simulink library "sm_trackV_lib_terrain_contact_s46"  (R2026a)
settings: Solver=VariableStepAuto
undefined symbols (not defined in the file): B1, B2, B3, B4, B5, B6, B7, B8, L1, L10, L11, L12, L13, L14, L15, L16, L17, L18, L19, L2, L20, L21, L22, L23, L24, L25, L26, L27, L28, L29, L3, L30, L31, L32, L33, L34, L35, L36, L37, L38, L39, L4, L40, L41, L42, L43, L44, L45, L46, L5, L6, L7, L8, L9, Road, Scene, X, Y, Z
libraries: sm_trackV_lib_terrain_contact_elem x92, $bdroot x22, sm_excv_scene_lib x5, sm_lib x4
Description:
  | Copyright 2024-2026 The MathWorks, Inc.
settings Model: Creator=smiller  LastModifiedBy=smiller

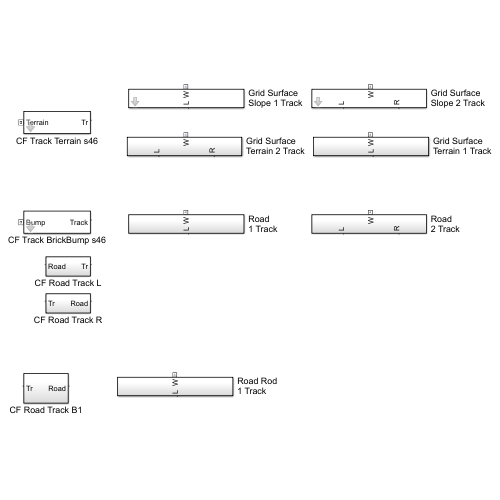
[thumbnail: Simulink's stored preview of the top-level diagram]
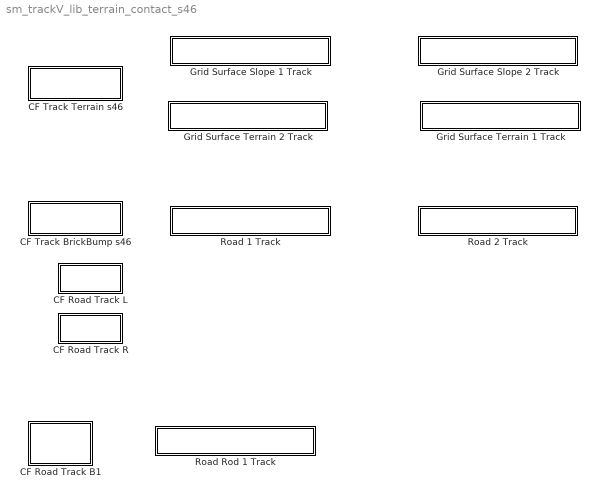
== system sm_trackV_lib_terrain_contact_s46 ==
  CF Road Track B1 : Subsystem
  CF Road Track L : Subsystem
  CF Road Track R : Subsystem
  CF Track BrickBump s46 : Subsystem  mask(Contact Forces, Full Track to Bump){K_BrickBump=Scene.Contact.BrickBump.K, B_BrickBump=Scene.Contact.BrickBump.B, TW_BrickBump=Scene.Contact.BrickBump.TW}
      mask prompts: K_BrickBump "Normal Stiffness (N/m)"; B_BrickBump "Normal Damping (N/(m/s))"; TW_BrickBump "Normal Transition Width (m)"
      mask help: Models contact force between all track segments and bump.
  CF Track Terrain s46 : Subsystem  mask(Contact Forces, Full Track to Terrain){K_Road=Scene.Contact.Terrain.K, B_Road=Scene.Contact.Terrain.B, TW_Road=Scene.Contact.Terrain.TW, F_dyn_Road=Scene.Contact.Terrain.mud, F_stat_Road=Scene.Contact.Terrain.mus, CV_Road=Scene.Contact.Terrain.CV}
      mask prompts: K_Road "Normal Stiffness (N/m)"; B_Road "Normal Damping (N/(m/s))"; TW_Road "Normal Transition Width (m)"; F_dyn_Road "Coefficient of Dynamic Friction"; F_stat_Road "Coefficient of Static Friction"; CV_Road "Critical Velocity (m/s)"
      mask help: Models contact force between all track segments and the terrain.
  Grid Surface Slope 1 Track : Subsystem  mask{road_len=Scene.Slope.road_len, road_wid=Scene.Slope.road_wid, slope_rise=Scene.Slope.slope_rise, slope_run=Scene.Slope.slope_run, slope_x0=Scene.Slope.slope_start, slope_xres=Scene.Slope.slope_xres, surface_clr=Scene.Slope.clr, surface_opc=Scene.Slope.opc, K_Road=Scene.Contact.Terrain.K, B_Road=Scene.Contact.Terrain.B, TW_Road=Scene.Contact.Terrain.TW, F_dyn_Road=Scene.Contact.Terrain.mud, F_stat_Road=Scene.Contact.Terrain.mus, CV_Road=Scene.Contact.Terrain.CV}
      mask prompts: road_len "Road Length (m)"; road_wid "Road Width (m)"; slope_rise "Slope Rise (m)"; slope_run "Slope Run(m)"; slope_x0 "Slope Start (m)"; slope_xres "Slope Resolution (m)"; surface_clr "Color [R G B] (0-1)"; surface_opc "Opacity (0-1)"; K_Road "Normal Stiffness (N/m)"; B_Road "Normal Damping (N/(m/s))"; TW_Road "Normal Transition Width (m)"; F_dyn_Road "Coefficient of Dynamic Friction"; F_stat_Road "Coefficient of Static Friction"; CV_Road "Critical Velocity (m/s)"
      mask TypeOptions road_len:
      | Grid Surface
      | Slope/road_len
      mask TypeOptions road_wid:
      | Grid Surface
      | Slope/road_wid
      mask TypeOptions slope_rise:
      | Grid Surface
      | Slope/slope_rise
      mask TypeOptions slope_run:
      | Grid Surface
      | Slope/slope_run
      mask TypeOptions slope_x0:
      | Grid Surface
      | Slope/slope_x0
      mask TypeOptions slope_xres:
      | Grid Surface
      | Slope/slope_xres
      mask TypeOptions surface_clr:
      | Grid Surface
      | Slope/surface_clr
      mask TypeOptions surface_opc:
      | Grid Surface
      | Slope/surface_opc
      mask TypeOptions K_Road: CF Track Terrain L/K_Road
      mask TypeOptions B_Road: CF Track Terrain L/B_Road
      mask TypeOptions TW_Road: CF Track Terrain L/TW_Road
      mask TypeOptions F_dyn_Road: CF Track Terrain L/F_dyn_Road
      mask TypeOptions F_stat_Road: CF Track Terrain L/F_stat_Road
      mask TypeOptions CV_Road: CF Track Terrain L/CV_Road
      mask DialogControl cont_slope Prompt: Slope
      mask DialogControl cont_contact Prompt: Contact
  Grid Surface Slope 2 Track : Subsystem  mask{road_len=Scene.Slope.road_len, road_wid=Scene.Slope.road_wid, slope_rise=Scene.Slope.slope_rise, slope_run=Scene.Slope.slope_run, slope_x0=Scene.Slope.slope_start, slope_xres=Scene.Slope.slope_xres, surface_clr=Scene.Slope.clr, surface_opc=Scene.Slope.opc, TW_Road=Scene.Contact.Terrain.TW, B_Road=Scene.Contact.Terrain.B, K_Road=Scene.Contact.Terrain.K, F_dyn_Road=Scene.Contact.Terrain.mud, F_stat_Road=Scene.Contact.Terrain.mus, CV_Road=Scene.Contact.Terrain.CV}
      mask prompts: road_len "Road Length (m)"; road_wid "Road Width (m)"; slope_rise "Slope Rise (m)"; slope_run "Slope Run(m)"; slope_x0 "Slope Start (m)"; slope_xres "Slope Resolution (m)"; surface_clr "Color [R G B] (0-1)"; surface_opc "Opacity (0-1)"; TW_Road "Normal Transition Width (m)"; B_Road "Normal Damping (N/(m/s))"; K_Road "Normal Stiffness (N/m)"; F_dyn_Road "Coefficient of Dynamic Friction"; F_stat_Road "Coefficient of Static Friction"; CV_Road "Critical Velocity (m/s)"
      mask TypeOptions road_len:
      | Grid Surface
      | Slope/road_len
      mask TypeOptions road_wid:
      | Grid Surface
      | Slope/road_wid
      mask TypeOptions slope_rise:
      | Grid Surface
      | Slope/slope_rise
      mask TypeOptions slope_run:
      | Grid Surface
      | Slope/slope_run
      mask TypeOptions slope_x0:
      | Grid Surface
      | Slope/slope_x0
      mask TypeOptions slope_xres:
      | Grid Surface
      | Slope/slope_xres
      mask TypeOptions surface_clr:
      | Grid Surface
      | Slope/surface_clr
      mask TypeOptions surface_opc:
      | Grid Surface
      | Slope/surface_opc
      mask TypeOptions TW_Road: CF Track Terrain L/TW_Road | CF Track Terrain R/TW_Road
      mask TypeOptions B_Road: CF Track Terrain L/B_Road | CF Track Terrain R/B_Road
      mask TypeOptions K_Road: CF Track Terrain L/K_Road | CF Track Terrain R/K_Road
      mask TypeOptions F_dyn_Road: CF Track Terrain L/F_dyn_Road | CF Track Terrain R/F_dyn_Road
      mask TypeOptions F_stat_Road: CF Track Terrain L/F_stat_Road | CF Track Terrain R/F_stat_Road
      mask TypeOptions CV_Road: CF Track Terrain L/CV_Road | CF Track Terrain R/CV_Road
      mask DialogControl cont_slope Prompt: Slope
      mask DialogControl cont_contact Prompt: Contact
  Grid Surface Terrain 1 Track : Subsystem
  Grid Surface Terrain 2 Track : Subsystem
  Road 1 Track : Subsystem
  Road 2 Track : Subsystem
  Road Rod 1 Track : Subsystem

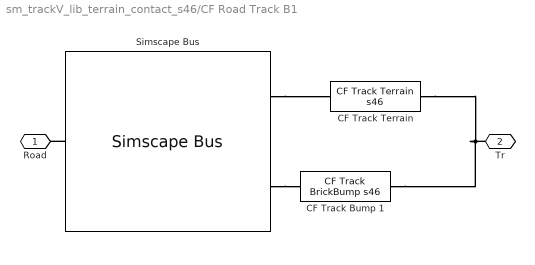
== system sm_trackV_lib_terrain_contact_s46/CF Road Track B1 ==
  CF Track Bump 1 : $bdroot/CF Track BrickBump s46  K_BrickBump=Scene.Contact.BrickBump.K  B_BrickBump=Scene.Contact.BrickBump.B  TW_BrickBump=Scene.Contact.BrickBump.TW
      settings: LibrarySourceBlock=sm_chain_drive_lib/CF_BrickBump_Full
  CF Track Terrain : $bdroot/CF Track Terrain s46  K_Road=Scene.Contact.Terrain.K  B_Road=Scene.Contact.Terrain.B  TW_Road=Scene.Contact.Terrain.TW  F_dyn_Road=Scene.Contact.Terrain.mud  F_stat_Road=Scene.Contact.Terrain.mus  CV_Road=Scene.Contact.Terrain.CV
      settings: LibrarySourceBlock=sm_chain_drive_lib/CF_Road_Full
  Simscape Bus : SimscapeBus  HierarchyStrings=Road;B1  ConnectionType=Bus: CBO_Road8
  Road : PMIOPort  Side=Left
  Tr : PMIOPort  Port=2  Side=Right
  connections:
  CF Track Terrain/RConn1 -- Tr/RConn1 -- CF Track Bump 1/RConn1
  Simscape Bus/RConn1 -- Road/RConn1
  Simscape Bus/LConn1 -- CF Track Terrain/LConn1
  Simscape Bus/LConn2 -- CF Track Bump 1/LConn1

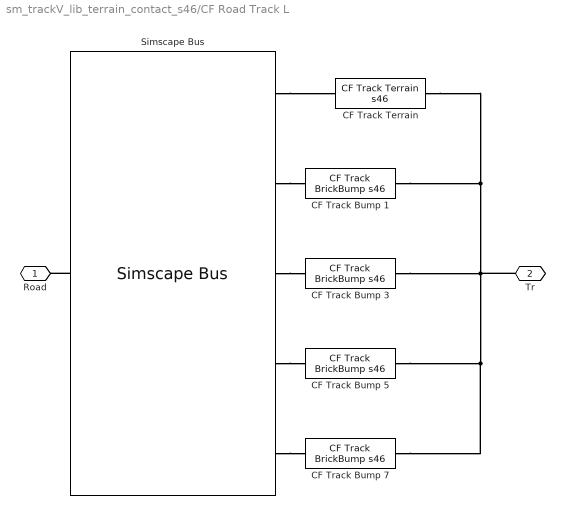
== system sm_trackV_lib_terrain_contact_s46/CF Road Track L ==
  CF Track Bump {1,3,5,7} (4 alike) : $bdroot/CF Track BrickBump s46  K_BrickBump=Scene.Contact.BrickBump.K  B_BrickBump=Scene.Contact.BrickBump.B  TW_BrickBump=Scene.Contact.BrickBump.TW
      settings: LibrarySourceBlock=sm_chain_drive_lib/CF_BrickBump_Full
  CF Track Terrain : $bdroot/CF Track Terrain s46  K_Road=Scene.Contact.Terrain.K  B_Road=Scene.Contact.Terrain.B  TW_Road=Scene.Contact.Terrain.TW  F_dyn_Road=Scene.Contact.Terrain.mud  F_stat_Road=Scene.Contact.Terrain.mus  CV_Road=Scene.Contact.Terrain.CV
      settings: LibrarySourceBlock=sm_chain_drive_lib/CF_Road_Full
  Simscape Bus : SimscapeBus  HierarchyStrings=Road;B1;B3;B5;B7  ConnectionType=Bus: CBO_Road8
  Road : PMIOPort  Side=Left
  Tr : PMIOPort  Port=2  Side=Right
  connections:
  Simscape Bus/LConn3 -- CF Track Bump 3/LConn1
  Simscape Bus/LConn2 -- CF Track Bump 1/LConn1
  Simscape Bus/LConn1 -- CF Track Terrain/LConn1
  Simscape Bus/RConn1 -- Road/RConn1
  Simscape Bus/LConn4 -- CF Track Bump 5/LConn1
  Simscape Bus/LConn5 -- CF Track Bump 7/LConn1
  CF Track Bump 1/RConn1 -- Tr/RConn1 -- CF Track Bump 7/RConn1 -- CF Track Bump 5/RConn1 -- CF Track Bump 3/RConn1 -- CF Track Terrain/RConn1

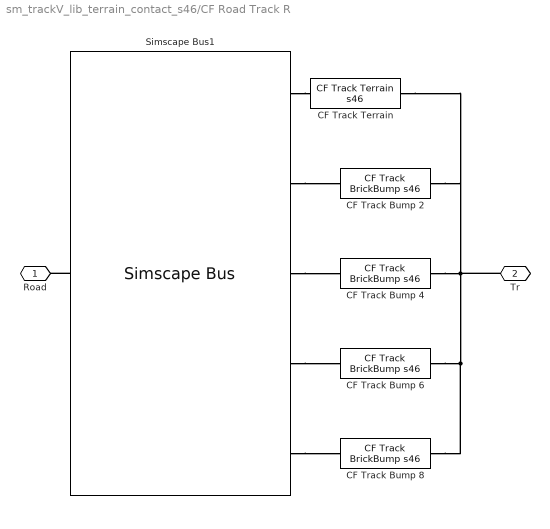
== system sm_trackV_lib_terrain_contact_s46/CF Road Track R ==
  CF Track Bump {2,4,6,8} (4 alike) : $bdroot/CF Track BrickBump s46  K_BrickBump=Scene.Contact.BrickBump.K  B_BrickBump=Scene.Contact.BrickBump.B  TW_BrickBump=Scene.Contact.BrickBump.TW
      settings: LibrarySourceBlock=sm_chain_drive_lib/CF_BrickBump_Full
  CF Track Terrain : $bdroot/CF Track Terrain s46  K_Road=Scene.Contact.Terrain.K  B_Road=Scene.Contact.Terrain.B  TW_Road=Scene.Contact.Terrain.TW  F_dyn_Road=Scene.Contact.Terrain.mud  F_stat_Road=Scene.Contact.Terrain.mus  CV_Road=Scene.Contact.Terrain.CV
      settings: LibrarySourceBlock=sm_chain_drive_lib/CF_Road_Full
  Simscape Bus1 : SimscapeBus  HierarchyStrings=Road;B2;B4;B6;B8  ConnectionType=Bus: CBO_Road8
  Road : PMIOPort  Side=Left
  Tr : PMIOPort  Port=2  Side=Right
  connections:
  CF Track Bump 6/RConn1 -- CF Track Bump 8/RConn1 -- CF Track Bump 4/RConn1 -- CF Track Bump 2/RConn1 -- CF Track Terrain/RConn1 -- Tr/RConn1
  Simscape Bus1/LConn5 -- CF Track Bump 8/LConn1
  Simscape Bus1/LConn4 -- CF Track Bump 6/LConn1
  Simscape Bus1/RConn1 -- Road/RConn1
  Simscape Bus1/LConn1 -- CF Track Terrain/LConn1
  Simscape Bus1/LConn2 -- CF Track Bump 2/LConn1
  Simscape Bus1/LConn3 -- CF Track Bump 4/LConn1

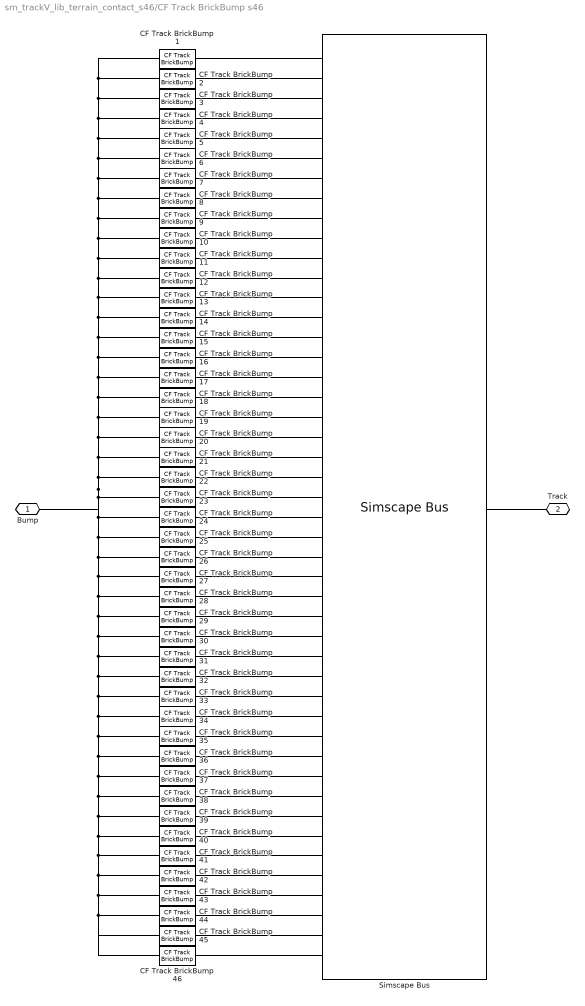
== system sm_trackV_lib_terrain_contact_s46/CF Track BrickBump s46 ==
  CF Track BrickBump {1..46} (46 alike) : sm_trackV_lib_terrain_contact_elem/CF Track BrickBump  NormalStiffness=K_BrickBump  NormalDamping=B_BrickBump  NormalTransitionRegionWidth=TW_BrickBump
      settings: LibrarySourceBlock=sm_chain_drive_lib/CF_BrickBump
  Simscape Bus : SimscapeBus  HierarchyStrings=L1;L2;L3;L4;L5;L6;L7;L8;L9;L10;L11;L12;L13;L14;L15;L16;L17;L18;L19;L20;L21;L22;L23;L24;L25;L26;L27;L28;L29;L30;L31;L32;L33;L34;L35;L36;L37;L38;L39;L40;L41;L42;L43;L44;L45;L46  ConnectionType=Bus: CBO_Chain46
  Bump : PMIOPort  Side=Left
  Track : PMIOPort  Port=2  Side=Right
  connections:
  CF Track BrickBump 1/LConn1 -- CF Track BrickBump 2/LConn1 -- CF Track BrickBump 3/LConn1 -- CF Track BrickBump 4/LConn1 -- CF Track BrickBump 5/LConn1 -- CF Track BrickBump 6/LConn1 -- CF Track BrickBump 7/LConn1 -- CF Track BrickBump 8/LConn1 -- CF Track BrickBump 9/LConn1 -- CF Track BrickBump 10/LConn1 -- CF Track BrickBump 11/LConn1 -- CF Track BrickBump 12/LConn1 -- CF Track BrickBump 13/LConn1 -- CF Track BrickBump 14/LConn1 -- CF Track BrickBump 15/LConn1 -- CF Track BrickBump 16/LConn1 -- Bump/RConn1 -- CF Track BrickBump 45/LConn1 -- CF Track BrickBump 46/LConn1 -- CF Track BrickBump 44/LConn1 -- CF Track BrickBump 43/LConn1 -- CF Track BrickBump 42/LConn1 -- CF Track BrickBump 41/LConn1 -- CF Track BrickBump 40/LConn1 -- CF Track BrickBump 39/LConn1 -- CF Track BrickBump 38/LConn1 -- CF Track BrickBump 37/LConn1 -- CF Track BrickBump 36/LConn1 -- CF Track BrickBump 35/LConn1 -- CF Track BrickBump 34/LConn1 -- CF Track BrickBump 33/LConn1 -- CF Track BrickBump 32/LConn1 -- CF Track BrickBump 31/LConn1 -- CF Track BrickBump 30/LConn1 -- CF Track BrickBump 29/LConn1 -- CF Track BrickBump 28/LConn1 -- CF Track BrickBump 27/LConn1 -- CF Track BrickBump 26/LConn1 -- CF Track BrickBump 25/LConn1 -- CF Track BrickBump 24/LConn1 -- CF Track BrickBump 23/LConn1 -- CF Track BrickBump 22/LConn1 -- CF Track BrickBump 21/LConn1 -- CF Track BrickBump 20/LConn1 -- CF Track BrickBump 19/LConn1 -- CF Track BrickBump 18/LConn1 -- CF Track BrickBump 17/LConn1
  Simscape Bus/RConn1 -- Track/RConn1
  CF Track BrickBump 1/RConn1 -- Simscape Bus/LConn1
  CF Track BrickBump 2/RConn1 -- Simscape Bus/LConn2
  CF Track BrickBump 4/RConn1 -- Simscape Bus/LConn4
  CF Track BrickBump 3/RConn1 -- Simscape Bus/LConn3
  CF Track BrickBump 5/RConn1 -- Simscape Bus/LConn5
  CF Track BrickBump 6/RConn1 -- Simscape Bus/LConn6
  CF Track BrickBump 7/RConn1 -- Simscape Bus/LConn7
  CF Track BrickBump 8/RConn1 -- Simscape Bus/LConn8
  CF Track BrickBump 9/RConn1 -- Simscape Bus/LConn9
  CF Track BrickBump 10/RConn1 -- Simscape Bus/LConn10
  CF Track BrickBump 11/RConn1 -- Simscape Bus/LConn11
  CF Track BrickBump 12/RConn1 -- Simscape Bus/LConn12
  CF Track BrickBump 13/RConn1 -- Simscape Bus/LConn13
  CF Track BrickBump 14/RConn1 -- Simscape Bus/LConn14
  CF Track BrickBump 15/RConn1 -- Simscape Bus/LConn15
  CF Track BrickBump 16/RConn1 -- Simscape Bus/LConn16
  CF Track BrickBump 17/RConn1 -- Simscape Bus/LConn17
  CF Track BrickBump 18/RConn1 -- Simscape Bus/LConn18
  CF Track BrickBump 19/RConn1 -- Simscape Bus/LConn19
  CF Track BrickBump 20/RConn1 -- Simscape Bus/LConn20
  CF Track BrickBump 21/RConn1 -- Simscape Bus/LConn21
  CF Track BrickBump 22/RConn1 -- Simscape Bus/LConn22
  CF Track BrickBump 23/RConn1 -- Simscape Bus/LConn23
  CF Track BrickBump 24/RConn1 -- Simscape Bus/LConn24
  CF Track BrickBump 25/RConn1 -- Simscape Bus/LConn25
  CF Track BrickBump 26/RConn1 -- Simscape Bus/LConn26
  CF Track BrickBump 27/RConn1 -- Simscape Bus/LConn27
  CF Track BrickBump 28/RConn1 -- Simscape Bus/LConn28
  CF Track BrickBump 29/RConn1 -- Simscape Bus/LConn29
  CF Track BrickBump 30/RConn1 -- Simscape Bus/LConn30
  CF Track BrickBump 31/RConn1 -- Simscape Bus/LConn31
  CF Track BrickBump 32/RConn1 -- Simscape Bus/LConn32
  CF Track BrickBump 33/RConn1 -- Simscape Bus/LConn33
  CF Track BrickBump 34/RConn1 -- Simscape Bus/LConn34
  CF Track BrickBump 35/RConn1 -- Simscape Bus/LConn35
  CF Track BrickBump 36/RConn1 -- Simscape Bus/LConn36
  CF Track BrickBump 37/RConn1 -- Simscape Bus/LConn37
  CF Track BrickBump 38/RConn1 -- Simscape Bus/LConn38
  CF Track BrickBump 39/RConn1 -- Simscape Bus/LConn39
  CF Track BrickBump 40/RConn1 -- Simscape Bus/LConn40
  CF Track BrickBump 41/RConn1 -- Simscape Bus/LConn41
  CF Track BrickBump 42/RConn1 -- Simscape Bus/LConn42
  CF Track BrickBump 43/RConn1 -- Simscape Bus/LConn43
  CF Track BrickBump 44/RConn1 -- Simscape Bus/LConn44
  CF Track BrickBump 45/RConn1 -- Simscape Bus/LConn45
  CF Track BrickBump 46/RConn1 -- Simscape Bus/LConn46

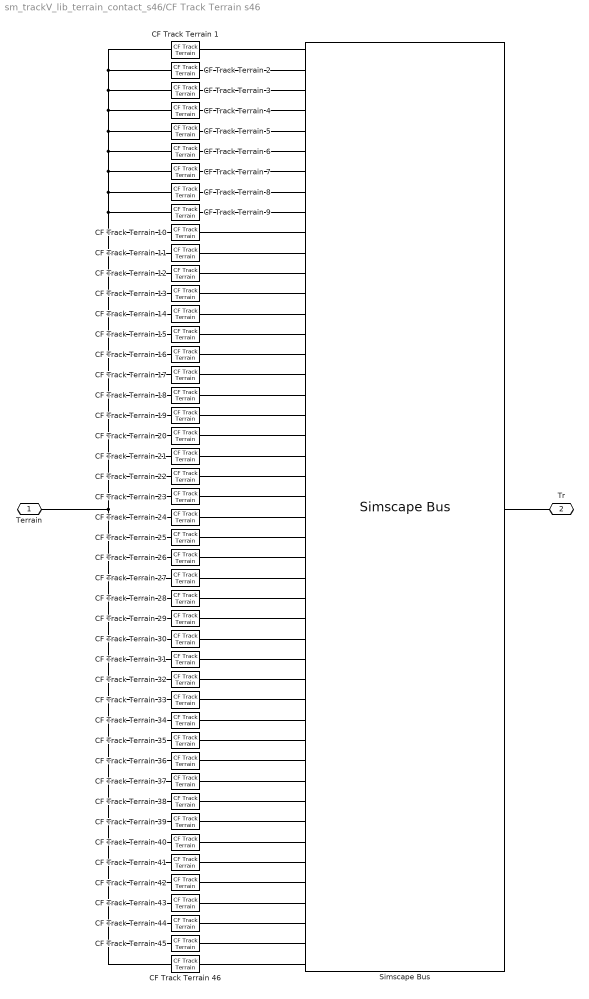
== system sm_trackV_lib_terrain_contact_s46/CF Track Terrain s46 ==
  CF Track Terrain {1..46} (46 alike) : sm_trackV_lib_terrain_contact_elem/CF Track Terrain  NormalStiffness=K_Road  NormalDamping=B_Road  NormalTransitionRegionWidth=TW_Road  CoefficientOfDynamicFriction=F_dyn_Road  CoefficientOfStaticFriction=F_stat_Road  FrictionalCriticalVelocity=CV_Road
      settings: LibrarySourceBlock=sm_chain_drive_lib/CF_Road
  Simscape Bus : SimscapeBus  HierarchyStrings=L1;L2;L3;L4;L5;L6;L7;L8;L9;L10;L11;L12;L13;L14;L15;L16;L17;L18;L19;L20;L21;L22;L23;L24;L25;L26;L27;L28;L29;L30;L31;L32;L33;L34;L35;L36;L37;L38;L39;L40;L41;L42;L43;L44;L45;L46  ConnectionType=Bus: CBO_Chain46
  Terrain : PMIOPort  Side=Left
  Tr : PMIOPort  Port=2  Side=Right
  connections:
  CF Track Terrain 46/RConn1 -- Simscape Bus/LConn46
  CF Track Terrain 45/RConn1 -- Simscape Bus/LConn45
  CF Track Terrain 44/RConn1 -- Simscape Bus/LConn44
  CF Track Terrain 43/RConn1 -- Simscape Bus/LConn43
  CF Track Terrain 42/RConn1 -- Simscape Bus/LConn42
  CF Track Terrain 41/RConn1 -- Simscape Bus/LConn41
  CF Track Terrain 40/RConn1 -- Simscape Bus/LConn40
  CF Track Terrain 39/RConn1 -- Simscape Bus/LConn39
  CF Track Terrain 38/RConn1 -- Simscape Bus/LConn38
  CF Track Terrain 37/RConn1 -- Simscape Bus/LConn37
  CF Track Terrain 36/RConn1 -- Simscape Bus/LConn36
  CF Track Terrain 35/RConn1 -- Simscape Bus/LConn35
  CF Track Terrain 34/RConn1 -- Simscape Bus/LConn34
  CF Track Terrain 33/RConn1 -- Simscape Bus/LConn33
  CF Track Terrain 32/RConn1 -- Simscape Bus/LConn32
  CF Track Terrain 31/RConn1 -- Simscape Bus/LConn31
  CF Track Terrain 30/RConn1 -- Simscape Bus/LConn30
  CF Track Terrain 29/RConn1 -- Simscape Bus/LConn29
  CF Track Terrain 28/RConn1 -- Simscape Bus/LConn28
  CF Track Terrain 27/RConn1 -- Simscape Bus/LConn27
  CF Track Terrain 26/RConn1 -- Simscape Bus/LConn26
  CF Track Terrain 25/RConn1 -- Simscape Bus/LConn25
  CF Track Terrain 24/RConn1 -- Simscape Bus/LConn24
  CF Track Terrain 23/RConn1 -- Simscape Bus/LConn23
  CF Track Terrain 22/RConn1 -- Simscape Bus/LConn22
  CF Track Terrain 21/RConn1 -- Simscape Bus/LConn21
  CF Track Terrain 20/RConn1 -- Simscape Bus/LConn20
  CF Track Terrain 19/RConn1 -- Simscape Bus/LConn19
  CF Track Terrain 18/RConn1 -- Simscape Bus/LConn18
  CF Track Terrain 17/RConn1 -- Simscape Bus/LConn17
  CF Track Terrain 16/RConn1 -- Simscape Bus/LConn16
  CF Track Terrain 15/RConn1 -- Simscape Bus/LConn15
  CF Track Terrain 14/RConn1 -- Simscape Bus/LConn14
  CF Track Terrain 13/RConn1 -- Simscape Bus/LConn13
  CF Track Terrain 12/RConn1 -- Simscape Bus/LConn12
  CF Track Terrain 11/RConn1 -- Simscape Bus/LConn11
  CF Track Terrain 10/RConn1 -- Simscape Bus/LConn10
  CF Track Terrain 9/RConn1 -- Simscape Bus/LConn9
  CF Track Terrain 8/RConn1 -- Simscape Bus/LConn8
  CF Track Terrain 7/RConn1 -- Simscape Bus/LConn7
  CF Track Terrain 6/RConn1 -- Simscape Bus/LConn6
  CF Track Terrain 5/RConn1 -- Simscape Bus/LConn5
  CF Track Terrain 3/RConn1 -- Simscape Bus/LConn3
  CF Track Terrain 4/RConn1 -- Simscape Bus/LConn4
  CF Track Terrain 2/RConn1 -- Simscape Bus/LConn2
  Simscape Bus/LConn1 -- CF Track Terrain 1/RConn1
  Simscape Bus/RConn1 -- Tr/RConn1
  CF Track Terrain 1/LConn1 -- CF Track Terrain 2/LConn1 -- CF Track Terrain 3/LConn1 -- CF Track Terrain 4/LConn1 -- CF Track Terrain 5/LConn1 -- CF Track Terrain 6/LConn1 -- CF Track Terrain 7/LConn1 -- CF Track Terrain 8/LConn1 -- CF Track Terrain 9/LConn1 -- CF Track Terrain 10/LConn1 -- CF Track Terrain 11/LConn1 -- CF Track Terrain 12/LConn1 -- CF Track Terrain 13/LConn1 -- CF Track Terrain 14/LConn1 -- CF Track Terrain 15/LConn1 -- CF Track Terrain 16/LConn1 -- CF Track Terrain 17/LConn1 -- CF Track Terrain 18/LConn1 -- CF Track Terrain 45/LConn1 -- CF Track Terrain 46/LConn1 -- CF Track Terrain 44/LConn1 -- CF Track Terrain 43/LConn1 -- CF Track Terrain 42/LConn1 -- CF Track Terrain 41/LConn1 -- CF Track Terrain 40/LConn1 -- CF Track Terrain 39/LConn1 -- CF Track Terrain 38/LConn1 -- CF Track Terrain 37/LConn1 -- CF Track Terrain 36/LConn1 -- CF Track Terrain 35/LConn1 -- CF Track Terrain 34/LConn1 -- CF Track Terrain 33/LConn1 -- CF Track Terrain 32/LConn1 -- CF Track Terrain 31/LConn1 -- CF Track Terrain 30/LConn1 -- CF Track Terrain 29/LConn1 -- CF Track Terrain 28/LConn1 -- CF Track Terrain 27/LConn1 -- CF Track Terrain 26/LConn1 -- CF Track Terrain 25/LConn1 -- CF Track Terrain 24/LConn1 -- Terrain/RConn1 -- CF Track Terrain 23/LConn1 -- CF Track Terrain 22/LConn1 -- CF Track Terrain 21/LConn1 -- CF Track Terrain 20/LConn1 -- CF Track Terrain 19/LConn1

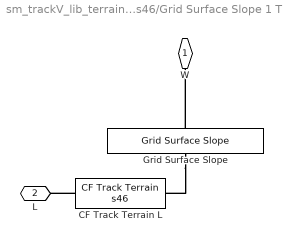
== system sm_trackV_lib_terrain_contact_s46/Grid Surface Slope 1 Track ==
  CF Track Terrain L : $bdroot/CF Track Terrain s46  K_Road=K_Road  B_Road=B_Road  TW_Road=TW_Road  F_dyn_Road=F_dyn_Road  F_stat_Road=F_stat_Road  CV_Road=CV_Road
      settings: LibrarySourceBlock=sm_chain_drive_lib/CF_Road_Full
  Grid Surface Slope : sm_excv_scene_lib/Grid Surface Slope  road_len=road_len  road_wid=road_wid  slope_run=slope_run  slope_rise=slope_rise  slope_x0=slope_x0  slope_xres=slope_xres  surface_clr=surface_clr  surface_opc=surface_opc
  W : PMIOPort  Side=Right
  L : PMIOPort  Port=2  Side=Left
  connections:
  Grid Surface Slope/LConn1 -- CF Track Terrain L/LConn1
  Grid Surface Slope/RConn1 -- W/RConn1
  CF Track Terrain L/RConn1 -- L/RConn1

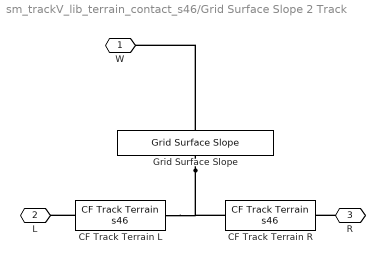
== system sm_trackV_lib_terrain_contact_s46/Grid Surface Slope 2 Track ==
  CF Track Terrain L : $bdroot/CF Track Terrain s46  K_Road=K_Road  B_Road=B_Road  TW_Road=TW_Road  F_dyn_Road=F_dyn_Road  F_stat_Road=F_stat_Road  CV_Road=CV_Road
      settings: LibrarySourceBlock=sm_chain_drive_lib/CF_Road_Full
  CF Track Terrain R : $bdroot/CF Track Terrain s46  K_Road=K_Road  B_Road=B_Road  TW_Road=TW_Road  F_dyn_Road=F_dyn_Road  F_stat_Road=F_stat_Road  CV_Road=CV_Road
      settings: LibrarySourceBlock=sm_chain_drive_lib/CF_Road_Full
  Grid Surface Slope : sm_excv_scene_lib/Grid Surface Slope  road_len=road_len  road_wid=road_wid  slope_run=slope_run  slope_rise=slope_rise  slope_x0=slope_x0  slope_xres=slope_xres  surface_clr=surface_clr  surface_opc=surface_opc
  W : PMIOPort  Side=Right
  L : PMIOPort  Port=2  Side=Left
  R : PMIOPort  Port=3  Side=Left
  connections:
  Grid Surface Slope/RConn1 -- W/RConn1
  CF Track Terrain L/RConn1 -- L/RConn1
  R/RConn1 -- CF Track Terrain R/RConn1
  Grid Surface Slope/LConn1 -- CF Track Terrain L/LConn1 -- CF Track Terrain R/LConn1

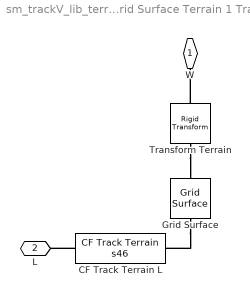
== system sm_trackV_lib_terrain_contact_s46/Grid Surface Terrain 1 Track ==
  CF Track Terrain L : $bdroot/CF Track Terrain s46  K_Road=Scene.Contact.Terrain.K  B_Road=Scene.Contact.Terrain.B  TW_Road=Scene.Contact.Terrain.TW  F_dyn_Road=Scene.Contact.Terrain.mud  F_stat_Road=Scene.Contact.Terrain.mus  CV_Road=Scene.Contact.Terrain.CV
      settings: LibrarySourceBlock=sm_chain_drive_lib/CF_Road_Full
  Grid Surface : sm_lib/Curves and Surfaces/Grid Surface  XGridVector=Scene.Terrain.xg  XGridVectorUnits=m  YGridVector=Scene.Terrain.yg  YGridVectorUnits=m  ZHeights=Scene.Terrain.z_heights_data  ZHeightsUnits=m  GraphicType=FromGeometry  GraphicVisPropType=SimpleVisualProperties  GraphicDiffuseColor=[0.8196 0.7255 0.5098]  GraphicOpacity=1.0  GraphicSpecularColor=[0.5 0.5 0.5 1.0]  GraphicAmbientColor=[0.15 0.15 0.15 1.0]  GraphicEmissiveColor=[0.0 0.0 0.0 1.0]  GraphicShininess=75
  Transform Terrain : sm_lib/Frames and Transforms/Rigid Transform  RotationMethod=None  FollAlignAxisA=+X  BaseAlignAxisA=+Y  FollAlignAxisB=+Y  BaseAlignAxisB=+Z  RotationStandardAxis=+Z  RotationAngle=0.0  RotationAngleUnits=deg  RotationArbitraryAxis=[0 0 1]  RotationSequenceAxes=FollowerAxes  RotationSequence=XYX  RotationSequenceAngles=[0 0 0]  RotationSequenceAnglesUnits=deg  RotationMatrix=[1 0 0; 0 1 0; 0 0 1]  Quaternion=[1 0 0 0]  TranslationMethod=Cartesian  TranslationCartesianOffset="[-45 -45+2.5  -2.75+0.2]"  TranslationCartesianOffsetUnits=m  TranslationStandardAxis=+Z  TranslationStandardOffset=0  TranslationStandardOffsetUnits=m  TranslationROffset=0  TranslationROffsetUnits=m  TranslationThetaOffset=0  TranslationThetaOffsetUnits=deg  TranslationZOffset=0  TranslationZOffsetUnits=m
  W : PMIOPort  Side=Right
  L : PMIOPort  Port=2  Side=Left
  connections:
  Transform Terrain/LConn1 -- W/RConn1
  Grid Surface/RConn1 -- CF Track Terrain L/LConn1
  Transform Terrain/RConn1 -- Grid Surface/LConn1
  CF Track Terrain L/RConn1 -- L/RConn1

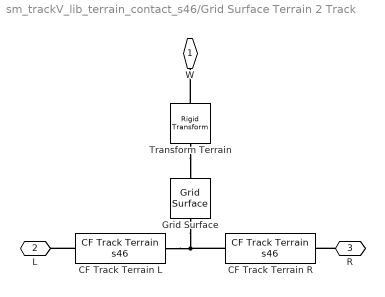
== system sm_trackV_lib_terrain_contact_s46/Grid Surface Terrain 2 Track ==
  CF Track Terrain L : $bdroot/CF Track Terrain s46  K_Road=Scene.Contact.Terrain.K  B_Road=Scene.Contact.Terrain.B  TW_Road=Scene.Contact.Terrain.TW  F_dyn_Road=Scene.Contact.Terrain.mud  F_stat_Road=Scene.Contact.Terrain.mus  CV_Road=Scene.Contact.Terrain.CV
      settings: LibrarySourceBlock=sm_chain_drive_lib/CF_Road_Full
  CF Track Terrain R : $bdroot/CF Track Terrain s46  K_Road=Scene.Contact.Terrain.K  B_Road=Scene.Contact.Terrain.B  TW_Road=Scene.Contact.Terrain.TW  F_dyn_Road=Scene.Contact.Terrain.mud  F_stat_Road=Scene.Contact.Terrain.mus  CV_Road=Scene.Contact.Terrain.CV
      settings: LibrarySourceBlock=sm_chain_drive_lib/CF_Road_Full
  Grid Surface : sm_lib/Curves and Surfaces/Grid Surface  XGridVector=Scene.Terrain.xg  XGridVectorUnits=m  YGridVector=Scene.Terrain.yg  YGridVectorUnits=m  ZHeights=Scene.Terrain.z_heights_data  ZHeightsUnits=m  GraphicType=FromGeometry  GraphicVisPropType=SimpleVisualProperties  GraphicDiffuseColor=[0.8196 0.7255 0.5098]  GraphicOpacity=1.0  GraphicSpecularColor=[0.5 0.5 0.5 1.0]  GraphicAmbientColor=[0.15 0.15 0.15 1.0]  GraphicEmissiveColor=[0.0 0.0 0.0 1.0]  GraphicShininess=75
  Transform Terrain : sm_lib/Frames and Transforms/Rigid Transform  RotationMethod=None  FollAlignAxisA=+X  BaseAlignAxisA=+Y  FollAlignAxisB=+Y  BaseAlignAxisB=+Z  RotationStandardAxis=+Z  RotationAngle=0.0  RotationAngleUnits=deg  RotationArbitraryAxis=[0 0 1]  RotationSequenceAxes=FollowerAxes  RotationSequence=XYX  RotationSequenceAngles=[0 0 0]  RotationSequenceAnglesUnits=deg  RotationMatrix=[1 0 0; 0 1 0; 0 0 1]  Quaternion=[1 0 0 0]  TranslationMethod=Cartesian  TranslationCartesianOffset="[-45 -45+2.5  -2.75+0.2]"  TranslationCartesianOffsetUnits=m  TranslationStandardAxis=+Z  TranslationStandardOffset=0  TranslationStandardOffsetUnits=m  TranslationROffset=0  TranslationROffsetUnits=m  TranslationThetaOffset=0  TranslationThetaOffsetUnits=deg  TranslationZOffset=0  TranslationZOffsetUnits=m
  W : PMIOPort  Side=Right
  L : PMIOPort  Port=2  Side=Left
  R : PMIOPort  Port=3  Side=Left
  connections:
  R/RConn1 -- CF Track Terrain R/RConn1
  CF Track Terrain L/RConn1 -- L/RConn1
  Transform Terrain/RConn1 -- Grid Surface/LConn1
  Grid Surface/RConn1 -- CF Track Terrain L/LConn1 -- CF Track Terrain R/LConn1
  Transform Terrain/LConn1 -- W/RConn1

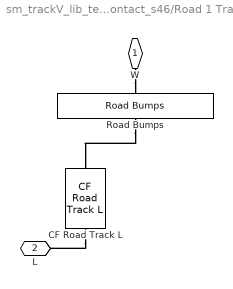
== system sm_trackV_lib_terrain_contact_s46/Road 1 Track ==
  CF Road Track L : $bdroot/CF Road Track L  SystemSampleTime=-1  VariantActivationTime=update diagram  EmptyChoice=off  PassThrough=off  PassThroughVariantControl=(default)  EmptyChoiceVariantControl=(default)  AllowFlexibleInterface=on  Latency=0  AutoFrameSizeCalculation=off
  Road Bumps : sm_excv_scene_lib/Road Bumps  road_x=Scene.Road.len  road_y=Scene.Road.wid  road_z=Scene.Road.hgt  bump_x=Scene.Road.Bump.len  bump_y=Scene.Road.Bump.wid  bump_z=Scene.Road.Bump.hgt  bloc_y=Scene.Road.Bump.offsety  bloc_z=Scene.Road.Bump.offsetz  bump_x0=Scene.Road.Bump.startx  bloc_dx=Scene.Road.Bump.deltax
  W : PMIOPort  Side=Right
  L : PMIOPort  Port=2  Side=Left
  connections:
  W/RConn1 -- Road Bumps/RConn1
  Road Bumps/LConn1 -- CF Road Track L/LConn1
  CF Road Track L/RConn1 -- L/RConn1

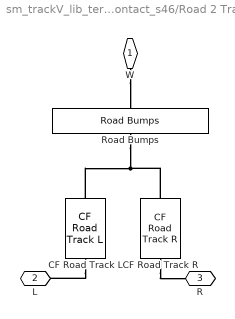
== system sm_trackV_lib_terrain_contact_s46/Road 2 Track ==
  CF Road Track L : $bdroot/CF Road Track L  SystemSampleTime=-1  VariantActivationTime=update diagram  EmptyChoice=off  PassThrough=off  PassThroughVariantControl=(default)  EmptyChoiceVariantControl=(default)  AllowFlexibleInterface=on  Latency=0  AutoFrameSizeCalculation=off
  CF Road Track R : $bdroot/CF Road Track R  SystemSampleTime=-1  VariantActivationTime=update diagram  EmptyChoice=off  PassThrough=off  PassThroughVariantControl=(default)  EmptyChoiceVariantControl=(default)  AllowFlexibleInterface=on  Latency=0  AutoFrameSizeCalculation=off
  Road Bumps : sm_excv_scene_lib/Road Bumps  road_x=Scene.Road.len  road_y=Scene.Road.wid  road_z=Scene.Road.hgt  bump_x=Scene.Road.Bump.len  bump_y=Scene.Road.Bump.wid  bump_z=Scene.Road.Bump.hgt  bloc_y=Scene.Road.Bump.offsety  bloc_z=Scene.Road.Bump.offsetz  bump_x0=Scene.Road.Bump.startx  bloc_dx=Scene.Road.Bump.deltax
  W : PMIOPort  Side=Right
  L : PMIOPort  Port=2  Side=Left
  R : PMIOPort  Port=3  Side=Left
  connections:
  W/RConn1 -- Road Bumps/RConn1
  CF Road Track R/RConn1 -- R/RConn1
  CF Road Track L/RConn1 -- L/RConn1
  CF Road Track R/LConn1 -- Road Bumps/LConn1 -- CF Road Track L/LConn1

== system sm_trackV_lib_terrain_contact_s46/Road Rod 1 Track ==
  CF Road Track L : $bdroot/CF Road Track B1  SystemSampleTime=-1  VariantActivationTime=update diagram  EmptyChoice=off  PassThrough=off  PassThroughVariantControl=(default)  EmptyChoiceVariantControl=(default)  AllowFlexibleInterface=on  Latency=0  AutoFrameSizeCalculation=off
  Road Rod : sm_excv_scene_lib/Road Rod  road_x=Scene.Road.len  road_y=Scene.Road.wid  road_z=Scene.Road.hgt  rod_len=Scene.Road.Rod.len  rod_rad=Scene.Road.Rod.rad  rod_y=Scene.Road.Rod.offsety  rod_z=Scene.Road.Rod.offsetz  rod_x0=Scene.Road.Rod.startx  rod_qz=Scene.Road.Rod.qz
  W : PMIOPort  Side=Right
  L : PMIOPort  Port=2  Side=Left
  connections:
  Road Rod/RConn1 -- W/RConn1
  CF Road Track L/LConn1 -- Road Rod/LConn1
  CF Road Track L/RConn1 -- L/RConn1
